simulink model "task2"  (R2012b)
settings: Solver=ode45  SolverMode=SingleTasking  StartTime=0.0  StopTime=10.0  RelTol=1e-3
settings Model: ExtModeTrigDuration=5000  Creator=yiwei.liu  LastModifiedBy=yiwei.liu
settings DataIOCC: SignalLoggingSaveFormat=ModelDataLogs
settings OptimizationCC: BlockReduction=off  BooleanDataType=off
settings DebuggingCC: SaveWithParameterizedLinksMsg=none  SignalResolutionControl=TryResolveAllWithWarning  SolverPrmCheckMsg=none  MultiTaskDSMMsg=warning  MultiTaskCondExecSysMsg=none  StrictBusMsg=None
settings HardwareCC: TargetUnknown=on
settings RTWCC: IncludeERTFirstTime=on

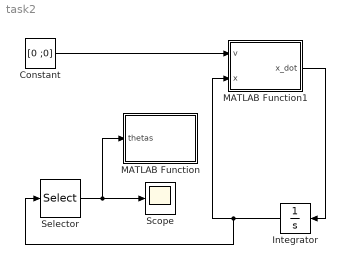
== system task2 ==
  Constant : Constant  Value=[0 ;0]
  Integrator : Integrator  InitialCondition=[0;0;0.1;0]
  MATLAB Function : MATLAB Function  TreatAsAtomicUnit=on
  MATLAB Function1 : MATLAB Function  TreatAsAtomicUnit=on
  Scope : Scope
  Selector : Selector  InputPortWidth=4  IndexOptions=Index vector (dialog)  Indices=[1 3]  OutputSizes=1
  wires:
  MATLAB Function1/1(x_dot) -> Integrator/1
  Integrator/1 -> MATLAB Function1/2(x), Selector/1
  Constant/1 -> MATLAB Function1/1(v)
  Selector/1 -> MATLAB Function/1(thetas), Scope/1

== matlab function task2/MATLAB Function ==
  data: thetas input
function  fcn(thetas)
%#codegen
A=[0 0 0 0 0];
B=[0 0 6 6 8];
C=[0 -1 -1 0 0];
D=[1 1 1 1 1];

A2=[0 0];
B2=[0 12];
C2=[0 0];
D2=[1 1];
L1=6;

L2=2;
%First Link

    theta1=thetas(1);
    theta2=thetas(2);
    newpoints=trans(theta1,A,B,C,D);
    p= (newpoints(1:1,1:5));

    q= (newpoints(2:2,1:5));

    r= (newpoints(3:3,1:5));
   % Second Link

    new2=trans2(theta2,L1,L2,A2,B2,C2,D2);
    %Frame 1 to frame 0
    x2= new2(1:1,1:2);
    y2= new2(2:2,1:2);
    z2= new2(3:3,1:2);

    new3 = trans(theta1,x2,y2,z2,D2);
    %ABC values of Link 2 in frame 0
    p2= (new3(1:1,1:2));

    q2= (new3(2:2,1:2));

    r2= (new3(3:3,1:2));
   
%     hold on;
    plot3(p,q,r,'-b*',p2,q2,r2,'-g*');
end

== matlab function task2/MATLAB Function1 ==
  data: v input; x_dot output; x input
function x_dot = fcn(v,x)
%#codegen
 
theta1= 0.03037;
theta2= 0.018143;
theta3= 0.18143;
theta4= 0.09213;
theta5= 0.6101;
theta6= 0.009673;

q1 = x(1);
q1_dot = x(2);
q2 = x(3);
q2_dot = x(4);
 
%v = [0 ; 0]
A = [theta1 + theta2*(sin(q2)^2) theta3*cos(q2) ; theta3*cos(q2) theta2];
B = [2*theta2*sin(q2)*cos(q2)*q2_dot (-1)*theta3*sin(q2)*q2_dot; (-1)*theta2*sin(q2)*cos(q2)*q1_dot  0];
C = [theta5*q1_dot ; theta6*q2_dot];
D = [0 ;(-1)*theta4*9.8*sin(q2)];
 
q_dd = [0;0];
q_dd = (A^(-1))*(v - B*[q1_dot ; q2_dot] - C - D) ;
q1_dd = q_dd(1);
q2_dd = q_dd(2);
x_dot = [q1_dot ;q1_dd ; q2_dot; q2_dd ]
 
end
